simulink model "CRH2forBenchmark_Copy"  (R2014a)
settings: Solver=ode3  StartTime=0.0  StopTime=1  FixedStep=1e-5  RelTol=1e-3
PostLoadFcn:
  | , if any(exist('dsrtsu_mdlpostloadfcn', 'file') == [2, 3, 6]), try dsrtsu_mdlpostloadfcn('Execute', bdroot); catch fprintf('Error in PostLoadFcn (dsrtsu_mdlpostloadfcn) for model "%s":\n %s\n', bdroot, lasterr); end, end,
values from neighbouring files (symbols this model uses):
  Cd = 0.016    [CRH2forBenchmark.mat]
  Lm = 0.032848    [CRH2forBenchmark.mat]
  Ln = 0.002    [CRH2forBenchmark.mat]
  Lr = 0.034142    [CRH2forBenchmark.mat]
  Ls = 0.0342654    [CRH2forBenchmark.mat]
  np = 2    [CRH2forBenchmark.mat]
  Rd = 6000    [CRH2forBenchmark.mat]
  Rn = 0.2    [CRH2forBenchmark.mat]
  Rr = 0.146    [CRH2forBenchmark.mat]
  Rs = 0.144    [CRH2forBenchmark.mat]
  ts = 1e-05    [CRH2forBenchmark.mat]
undefined symbols (not defined in the file): J, KIM, KIT, KPM, KPT, phir, Ts, Vge
libraries: simulink x20
(part 2 of 5)

== system CRH2forBenchmark_Copy/Benchmark/MFI1 ==
  MFI1 : Subsystem  mask(MFI){FaultType=Normal, FaultInjectionTime=1, FS=[128.7,0.038], Severity1=0.5, Severity3=0.2, Severity2=0.2, BearingFP=[1,8,25,25,65,0,20], NoiseSelec=off, NoiseFault=[0.001 1e-5 23341], AddMux=Add}
      mask prompts: FaultType "Fault Type"; FaultInjectionTime "Fault Injection Time(Step time)"; FS "Fundamental Frequency and Slip Ratio[f1 S]"; Severity1 "Mechanical Fault Severity (0-1)(Bar Broken fault;End Link Fault;Bearing Fault)"; Severity3 "Electrical Fault Severity(0-1)(Air Gap Eccentricity Fault)"; Severity2 "Insulation Fault Severity(0-1)(Inter-turn Short Circuit Fault)"; BearingFP "Bearing Fault Parameters [T Z fr d D a fcage]"; NoiseSelec "Noise Disturbance"; NoiseFault "Noise Disturbance(Noise power,Sample time,Seed)"; AddMux "Add or Mux(outside signal)"
      mask help:
      | Machine Fault Injector (MFI)
      | 1.Fault Injection Time:Set the parameter of Fault-Inject Time;
      | 2.Fundamental Frequency and Slip Ratio[f1 S]:The current frequency of motor stator and the motor Slip Ratio.
      | 3.Mechanical Fault Severity (0-1)(Bar Broken fault;End Link Fault;Bearing Fault):Mechanical Failure factor denotes the fault severity（0-1）.Three types of Mechanical faults are taken into consideration;
      | 4.Electrical Fault Severity(0-1)(Air Gap Eccentricity Fault):Electrical Failure factor denotes the fault severity（0-1）.
      | 5.Insulation Fault Severity(0-1)(Inter-turn Short Circuit Fault):Insulation Failure factor denotes the fault severity（0-1）.
      | 6.Bearing Fault Parameters [T Z fr d D a fcage]: The value of S are constraint to [1,2,3], T=1 represents the outer ring fault,T=2 represents the bearing inner race fault, T=3 represents rolling body defect fault;Z is the number of bearing rollers;fr is motor bearing frequency;d is the bearing diameter of the rolling body;D is bearing section diameter;a is contact angle;fcage is cage rotation frequency.
      mask TypeOptions FaultType: Normal | Bar Broken Fault | Inter-turn Short Circuit Fault | Air Gap Eccentricity Fault | End Link Fault | Bearing Fault | Outside Signal
      mask TypeOptions AddMux: Add | Mux | Replace
      mask Display: fprintf('Motor Fault Injection')
  MFI2 : Subsystem  mask(MFI){FaultType=Normal, FaultInjectionTime=1, FS=[128.7,0.038], Severity1=0.5, Severity3=0.2, Severity2=0.2, BearingFP=[1,8,25,25,65,0,20], NoiseSelec=off, NoiseFault=[0.001 1e-5 23341], AddMux=Add}
      mask prompts: FaultType "Fault Type"; FaultInjectionTime "Fault Injection Time(Step time)"; FS "Fundamental Frequency and Slip Ratio[f1 S]"; Severity1 "Mechanical Fault Severity (0-1)(Bar Broken fault;End Link Fault;Bearing Fault)"; Severity3 "Electrical Fault Severity(0-1)(Air Gap Eccentricity Fault)"; Severity2 "Insulation Fault Severity(0-1)(Inter-turn Short Circuit Fault)"; BearingFP "Bearing Fault Parameters [T Z fr d D a fcage]"; NoiseSelec "Noise Disturbance"; NoiseFault "Noise Disturbance(Noise power,Sample time,Seed)"; AddMux "Add or Mux(outside signal)"
      mask help:
      | Machine Fault Injector (MFI)
      | 1.Fault Injection Time:Set the parameter of Fault-Inject Time;
      | 2.Fundamental Frequency and Slip Ratio[f1 S]:The current frequency of motor stator and the motor Slip Ratio.
      | 3.Mechanical Fault Severity (0-1)(Bar Broken fault;End Link Fault;Bearing Fault):Mechanical Failure factor denotes the fault severity（0-1）.Three types of Mechanical faults are taken into consideration;
      | 4.Electrical Fault Severity(0-1)(Air Gap Eccentricity Fault):Electrical Failure factor denotes the fault severity（0-1）.
      | 5.Insulation Fault Severity(0-1)(Inter-turn Short Circuit Fault):Insulation Failure factor denotes the fault severity（0-1）.
      | 6.Bearing Fault Parameters [T Z fr d D a fcage]: The value of S are constraint to [1,2,3], T=1 represents the outer ring fault,T=2 represents the bearing inner race fault, T=3 represents rolling body defect fault;Z is the number of bearing rollers;fr is motor bearing frequency;d is the bearing diameter of the rolling body;D is bearing section diameter;a is contact angle;fcage is cage rotation frequency.
      mask TypeOptions FaultType: Normal | Bar Broken Fault | Inter-turn Short Circuit Fault | Air Gap Eccentricity Fault | End Link Fault | Bearing Fault | Outside Signal
      mask TypeOptions AddMux: Add | Mux | Replace
      mask Display: fprintf('Motor Fault Injection')
  MFI3 : Subsystem  mask(MFI){FaultType=Normal, FaultInjectionTime=1, FS=[128.7,0.038], Severity1=0.5, Severity3=0.2, Severity2=0.2, BearingFP=[1,8,25,25,65,0,20], NoiseSelec=off, NoiseFault=[0.001 1e-5 23341], AddMux=Add}
      mask prompts: FaultType "Fault Type"; FaultInjectionTime "Fault Injection Time(Step time)"; FS "Fundamental Frequency and Slip Ratio[f1 S]"; Severity1 "Mechanical Fault Severity (0-1)(Bar Broken fault;End Link Fault;Bearing Fault)"; Severity3 "Electrical Fault Severity(0-1)(Air Gap Eccentricity Fault)"; Severity2 "Insulation Fault Severity(0-1)(Inter-turn Short Circuit Fault)"; BearingFP "Bearing Fault Parameters [T Z fr d D a fcage]"; NoiseSelec "Noise Disturbance"; NoiseFault "Noise Disturbance(Noise power,Sample time,Seed)"; AddMux "Add or Mux(outside signal)"
      mask help:
      | Machine Fault Injector (MFI)
      | 1.Fault Injection Time:Set the parameter of Fault-Inject Time;
      | 2.Fundamental Frequency and Slip Ratio[f1 S]:The current frequency of motor stator and the motor Slip Ratio.
      | 3.Mechanical Fault Severity (0-1)(Bar Broken fault;End Link Fault;Bearing Fault):Mechanical Failure factor denotes the fault severity（0-1）.Three types of Mechanical faults are taken into consideration;
      | 4.Electrical Fault Severity(0-1)(Air Gap Eccentricity Fault):Electrical Failure factor denotes the fault severity（0-1）.
      | 5.Insulation Fault Severity(0-1)(Inter-turn Short Circuit Fault):Insulation Failure factor denotes the fault severity（0-1）.
      | 6.Bearing Fault Parameters [T Z fr d D a fcage]: The value of S are constraint to [1,2,3], T=1 represents the outer ring fault,T=2 represents the bearing inner race fault, T=3 represents rolling body defect fault;Z is the number of bearing rollers;fr is motor bearing frequency;d is the bearing diameter of the rolling body;D is bearing section diameter;a is contact angle;fcage is cage rotation frequency.
      mask TypeOptions FaultType: Normal | Bar Broken Fault | Inter-turn Short Circuit Fault | Air Gap Eccentricity Fault | End Link Fault | Bearing Fault | Outside Signal
      mask TypeOptions AddMux: Add | Mux | Replace
      mask Display: fprintf('Motor Fault Injection')
  MFI4 : Subsystem  mask(MFI){FaultType=Normal, FaultInjectionTime=1, FS=[128.7,0.038], Severity1=0.5, Severity3=0.2, Severity2=0.2, BearingFP=[1,8,25,25,65,0,20], NoiseSelec=off, NoiseFault=[0.001 1e-5 23341], AddMux=Add}
      mask prompts: FaultType "Fault Type"; FaultInjectionTime "Fault Injection Time(Step time)"; FS "Fundamental Frequency and Slip Ratio[f1 S]"; Severity1 "Mechanical Fault Severity (0-1)(Bar Broken fault;End Link Fault;Bearing Fault)"; Severity3 "Electrical Fault Severity(0-1)(Air Gap Eccentricity Fault)"; Severity2 "Insulation Fault Severity(0-1)(Inter-turn Short Circuit Fault)"; BearingFP "Bearing Fault Parameters [T Z fr d D a fcage]"; NoiseSelec "Noise Disturbance"; NoiseFault "Noise Disturbance(Noise power,Sample time,Seed)"; AddMux "Add or Mux(outside signal)"
      mask help:
      | Machine Fault Injector (MFI)
      | 1.Fault Injection Time:Set the parameter of Fault-Inject Time;
      | 2.Fundamental Frequency and Slip Ratio[f1 S]:The current frequency of motor stator and the motor Slip Ratio.
      | 3.Mechanical Fault Severity (0-1)(Bar Broken fault;End Link Fault;Bearing Fault):Mechanical Failure factor denotes the fault severity（0-1）.Three types of Mechanical faults are taken into consideration;
      | 4.Electrical Fault Severity(0-1)(Air Gap Eccentricity Fault):Electrical Failure factor denotes the fault severity（0-1）.
      | 5.Insulation Fault Severity(0-1)(Inter-turn Short Circuit Fault):Insulation Failure factor denotes the fault severity（0-1）.
      | 6.Bearing Fault Parameters [T Z fr d D a fcage]: The value of S are constraint to [1,2,3], T=1 represents the outer ring fault,T=2 represents the bearing inner race fault, T=3 represents rolling body defect fault;Z is the number of bearing rollers;fr is motor bearing frequency;d is the bearing diameter of the rolling body;D is bearing section diameter;a is contact angle;fcage is cage rotation frequency.
      mask TypeOptions FaultType: Normal | Bar Broken Fault | Inter-turn Short Circuit Fault | Air Gap Eccentricity Fault | End Link Fault | Bearing Fault | Outside Signal
      mask TypeOptions AddMux: Add | Mux | Replace
      mask Display: fprintf('Motor Fault Injection')
  MFI5 : Subsystem  mask(MFI){FaultType=Normal, FaultInjectionTime=1, FS=[128.7,0.038], Severity1=0.5, Severity3=0.2, Severity2=0.2, BearingFP=[1,8,25,25,65,0,20], NoiseSelec=off, NoiseFault=[0.001 1e-5 23341], AddMux=Add}
      mask prompts: FaultType "Fault Type"; FaultInjectionTime "Fault Injection Time(Step time)"; FS "Fundamental Frequency and Slip Ratio[f1 S]"; Severity1 "Mechanical Fault Severity (0-1)(Bar Broken fault;End Link Fault;Bearing Fault)"; Severity3 "Electrical Fault Severity(0-1)(Air Gap Eccentricity Fault)"; Severity2 "Insulation Fault Severity(0-1)(Inter-turn Short Circuit Fault)"; BearingFP "Bearing Fault Parameters [T Z fr d D a fcage]"; NoiseSelec "Noise Disturbance"; NoiseFault "Noise Disturbance(Noise power,Sample time,Seed)"; AddMux "Add or Mux(outside signal)"
      mask help:
      | Machine Fault Injector (MFI)
      | 1.Fault Injection Time:Set the parameter of Fault-Inject Time;
      | 2.Fundamental Frequency and Slip Ratio[f1 S]:The current frequency of motor stator and the motor Slip Ratio.
      | 3.Mechanical Fault Severity (0-1)(Bar Broken fault;End Link Fault;Bearing Fault):Mechanical Failure factor denotes the fault severity（0-1）.Three types of Mechanical faults are taken into consideration;
      | 4.Electrical Fault Severity(0-1)(Air Gap Eccentricity Fault):Electrical Failure factor denotes the fault severity（0-1）.
      | 5.Insulation Fault Severity(0-1)(Inter-turn Short Circuit Fault):Insulation Failure factor denotes the fault severity（0-1）.
      | 6.Bearing Fault Parameters [T Z fr d D a fcage]: The value of S are constraint to [1,2,3], T=1 represents the outer ring fault,T=2 represents the bearing inner race fault, T=3 represents rolling body defect fault;Z is the number of bearing rollers;fr is motor bearing frequency;d is the bearing diameter of the rolling body;D is bearing section diameter;a is contact angle;fcage is cage rotation frequency.
      mask TypeOptions FaultType: Normal | Bar Broken Fault | Inter-turn Short Circuit Fault | Air Gap Eccentricity Fault | End Link Fault | Bearing Fault | Outside Signal
      mask TypeOptions AddMux: Add | Mux | Replace
      mask Display: fprintf('Motor Fault Injection')
  MFI6 : Subsystem  mask(MFI){FaultType=Normal, FaultInjectionTime=1, FS=[128.7,0.038], Severity1=0.5, Severity3=0.2, Severity2=0.2, BearingFP=[1,8,25,25,65,0,20], NoiseSelec=off, NoiseFault=[0.001 1e-5 23341], AddMux=Add}
      mask prompts: FaultType "Fault Type"; FaultInjectionTime "Fault Injection Time(Step time)"; FS "Fundamental Frequency and Slip Ratio[f1 S]"; Severity1 "Mechanical Fault Severity (0-1)(Bar Broken fault;End Link Fault;Bearing Fault)"; Severity3 "Electrical Fault Severity(0-1)(Air Gap Eccentricity Fault)"; Severity2 "Insulation Fault Severity(0-1)(Inter-turn Short Circuit Fault)"; BearingFP "Bearing Fault Parameters [T Z fr d D a fcage]"; NoiseSelec "Noise Disturbance"; NoiseFault "Noise Disturbance(Noise power,Sample time,Seed)"; AddMux "Add or Mux(outside signal)"
      mask help:
      | Machine Fault Injector (MFI)
      | 1.Fault Injection Time:Set the parameter of Fault-Inject Time;
      | 2.Fundamental Frequency and Slip Ratio[f1 S]:The current frequency of motor stator and the motor Slip Ratio.
      | 3.Mechanical Fault Severity (0-1)(Bar Broken fault;End Link Fault;Bearing Fault):Mechanical Failure factor denotes the fault severity（0-1）.Three types of Mechanical faults are taken into consideration;
      | 4.Electrical Fault Severity(0-1)(Air Gap Eccentricity Fault):Electrical Failure factor denotes the fault severity（0-1）.
      | 5.Insulation Fault Severity(0-1)(Inter-turn Short Circuit Fault):Insulation Failure factor denotes the fault severity（0-1）.
      | 6.Bearing Fault Parameters [T Z fr d D a fcage]: The value of S are constraint to [1,2,3], T=1 represents the outer ring fault,T=2 represents the bearing inner race fault, T=3 represents rolling body defect fault;Z is the number of bearing rollers;fr is motor bearing frequency;d is the bearing diameter of the rolling body;D is bearing section diameter;a is contact angle;fcage is cage rotation frequency.
      mask TypeOptions FaultType: Normal | Bar Broken Fault | Inter-turn Short Circuit Fault | Air Gap Eccentricity Fault | End Link Fault | Bearing Fault | Outside Signal
      mask TypeOptions AddMux: Add | Mux | Replace
      mask Display: fprintf('Motor Fault Injection')

== system CRH2forBenchmark_Copy/Benchmark/SFI1 ==
  Normal : Inport
  Outside Signal : Inport  Port=2
  Subsystem : Subsystem
  Out : Outport
  wires:
  Normal/1 -> Subsystem/1(Normal)
  Outside Signal/1 -> Subsystem/2(Outside Signal)
  Subsystem/1(Out) -> Out/1

== system CRH2forBenchmark_Copy/Benchmark/SFI2 ==
  Normal : Inport
  Outside Signal : Inport  Port=2
  Subsystem : Subsystem
  Out : Outport
  wires:
  Normal/1 -> Subsystem/1(Normal)
  Outside Signal/1 -> Subsystem/2(Outside Signal)
  Subsystem/1(Out) -> Out/1

== system CRH2forBenchmark_Copy/Benchmark/TFI1 ==
  Nomal : Inport
  Outside Signal : Inport  Port=2
  TFI1Sub : Subsystem
  Out : Outport
  wires:
  Nomal/1 -> TFI1Sub/1(Nomal)
  Outside Signal/1 -> TFI1Sub/2(Outside Signal)
  TFI1Sub/1(Out) -> Out/1

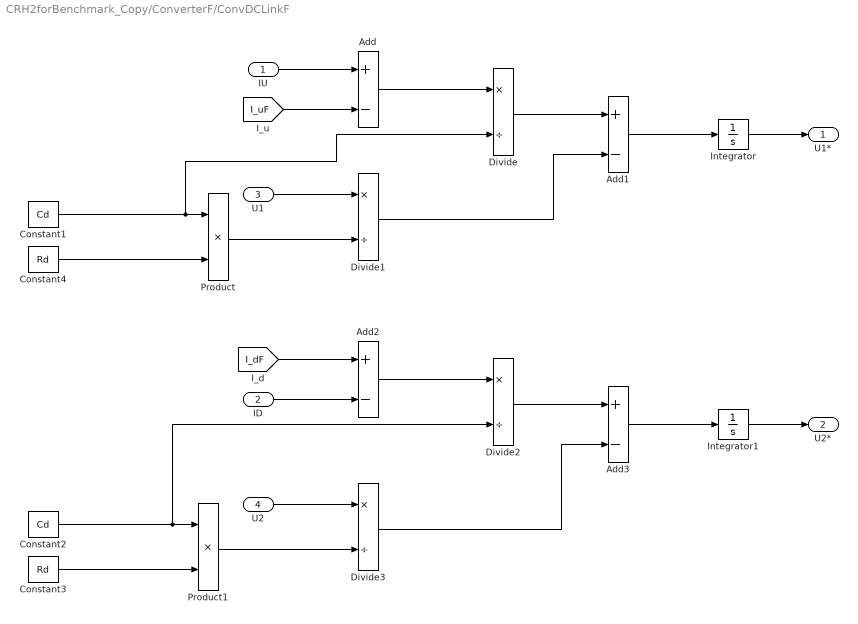
== system CRH2forBenchmark_Copy/ConverterF/ConvDCLinkF ==
  IU : Inport
  ID : Inport  Port=2
  U1 : Inport  Port=3
  U2 : Inport  Port=4
  Add{,1..3} (4 alike) : Sum  Inputs=+-  SampleTime=ts
  Constant1 : Constant  Value=Cd
  Constant2 : Constant  Value=Cd
  Constant3 : Constant  Value=Rd
  Constant4 : Constant  Value=Rd
  Divide{,1..3} (4 alike) : Product  Inputs=*/
  Integrator : Integrator
  Integrator1 : Integrator
  Product : Product  SampleTime=ts
  Product1 : Product  SampleTime=ts
  U1* : Outport
  U2* : Outport  Port=2
  wires:
  Add3/1 -> Integrator1/1
  Divide3/1 -> Add3/2
  Divide2/1 -> Add3/1
  U2/1 -> Divide3/1
  Product1/1 -> Divide3/2
  Add2/1 -> Divide2/1
  Constant2/1 -> Divide2/2, Product1/1
  [I_dF] -> Add2/1
  ID/1 -> Add2/2
  Add1/1 -> Integrator/1
  Divide1/1 -> Add1/2
  Divide/1 -> Add1/1
  U1/1 -> Divide1/1
  Constant1/1 -> Product/1, Divide/2
  Add/1 -> Divide/1
  [I_uF] -> Add/2
  IU/1 -> Add/1
  Integrator/1 -> U1*/1
  Integrator1/1 -> U2*/1
  Product/1 -> Divide1/2
  Constant4/1 -> Product/2
  Constant3/1 -> Product1/2

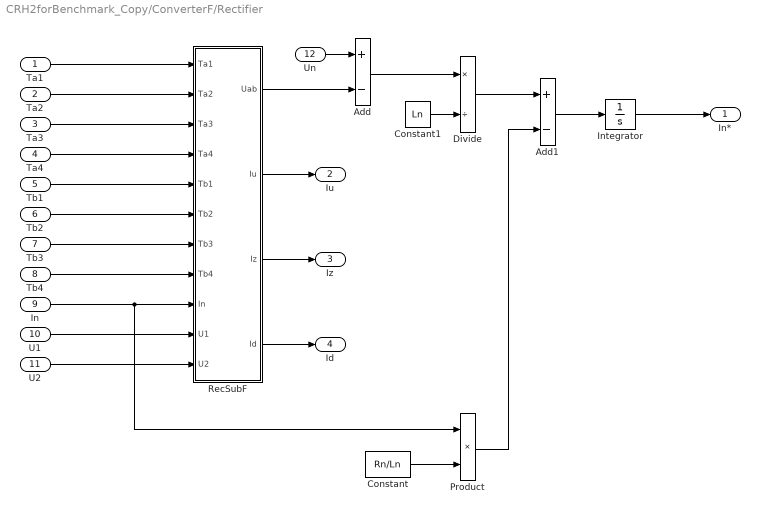
== system CRH2forBenchmark_Copy/ConverterF/Rectifier ==
  Ta1 : Inport
  Ta2 : Inport  Port=2
  Ta3 : Inport  Port=3
  Ta4 : Inport  Port=4
  Tb1 : Inport  Port=5
  Tb2 : Inport  Port=6
  Tb3 : Inport  Port=7
  Tb4 : Inport  Port=8
  In : Inport  Port=9
  U1 : Inport  Port=10
  U2 : Inport  Port=11
  Un : Inport  Port=12
  Add : Sum  Inputs=+-  SampleTime=ts
  Add1 : Sum  Inputs=+-  SampleTime=ts
  Constant : Constant  Value=Rn/Ln
  Constant1 : Constant  Value=Ln
  Divide : Product  Inputs=*/  SampleTime=ts
  Integrator : Integrator
  Product : Product  SampleTime=ts
  RecSubF : Subsystem
  In* : Outport
  Iu : Outport  Port=2
  Iz : Outport  Port=3
  Id : Outport  Port=4
  wires:
  RecSubF/4(Id) -> Id/1
  RecSubF/3(Iz) -> Iz/1
  RecSubF/2(Iu) -> Iu/1
  Tb2/1 -> RecSubF/6(Tb2)
  Ta3/1 -> RecSubF/3(Ta3)
  Un/1 -> Add/1
  Tb1/1 -> RecSubF/5(Tb1)
  Tb4/1 -> RecSubF/8(Tb4)
  Tb3/1 -> RecSubF/7(Tb3)
  In/1 -> Product/1, RecSubF/9(In)
  Ta4/1 -> RecSubF/4(Ta4)
  Ta2/1 -> RecSubF/2(Ta2)
  U2/1 -> RecSubF/11(U2)
  Integrator/1 -> In*/1
  Divide/1 -> Add1/1
  U1/1 -> RecSubF/10(U1)
  Constant/1 -> Product/2
  RecSubF/1(Uab) -> Add/2
  Ta1/1 -> RecSubF/1(Ta1)
  Add1/1 -> Integrator/1
  Product/1 -> Add1/2
  Constant1/1 -> Divide/2
  Add/1 -> Divide/1

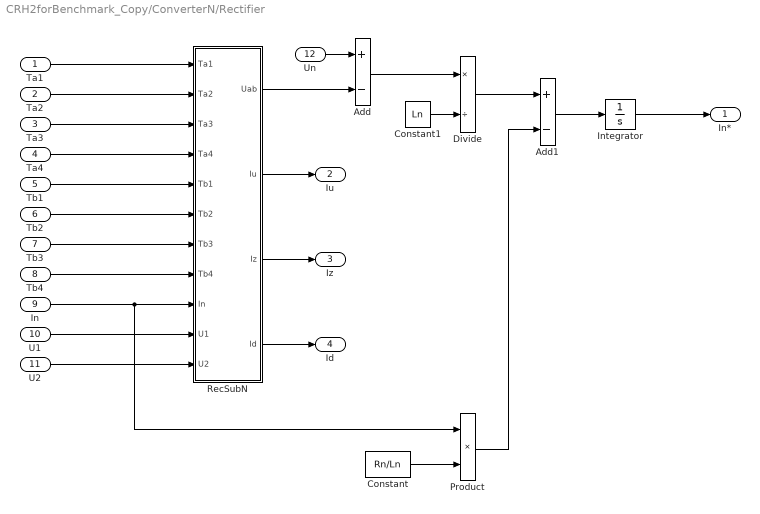
== system CRH2forBenchmark_Copy/ConverterN/Rectifier ==
  Ta1 : Inport
  Ta2 : Inport  Port=2
  Ta3 : Inport  Port=3
  Ta4 : Inport  Port=4
  Tb1 : Inport  Port=5
  Tb2 : Inport  Port=6
  Tb3 : Inport  Port=7
  Tb4 : Inport  Port=8
  In : Inport  Port=9
  U1 : Inport  Port=10
  U2 : Inport  Port=11
  Un : Inport  Port=12
  Add : Sum  Inputs=+-  SampleTime=ts
  Add1 : Sum  Inputs=+-  SampleTime=ts
  Constant : Constant  Value=Rn/Ln
  Constant1 : Constant  Value=Ln
  Divide : Product  Inputs=*/  SampleTime=ts
  Integrator : Integrator
  Product : Product  SampleTime=ts
  RecSubN : Subsystem
  In* : Outport
  Iu : Outport  Port=2
  Iz : Outport  Port=3
  Id : Outport  Port=4
  wires:
  Add/1 -> Divide/1
  Constant1/1 -> Divide/2
  Product/1 -> Add1/2
  Add1/1 -> Integrator/1
  Ta1/1 -> RecSubN/1(Ta1)
  RecSubN/1(Uab) -> Add/2
  Constant/1 -> Product/2
  U1/1 -> RecSubN/10(U1)
  Divide/1 -> Add1/1
  Integrator/1 -> In*/1
  U2/1 -> RecSubN/11(U2)
  Ta2/1 -> RecSubN/2(Ta2)
  Ta4/1 -> RecSubN/4(Ta4)
  In/1 -> RecSubN/9(In), Product/1
  Tb3/1 -> RecSubN/7(Tb3)
  Tb4/1 -> RecSubN/8(Tb4)
  Tb1/1 -> RecSubN/5(Tb1)
  Un/1 -> Add/1
  Ta3/1 -> RecSubN/3(Ta3)
  Tb2/1 -> RecSubN/6(Tb2)
  RecSubN/2(Iu) -> Iu/1
  RecSubN/3(Iz) -> Iz/1
  RecSubN/4(Id) -> Id/1

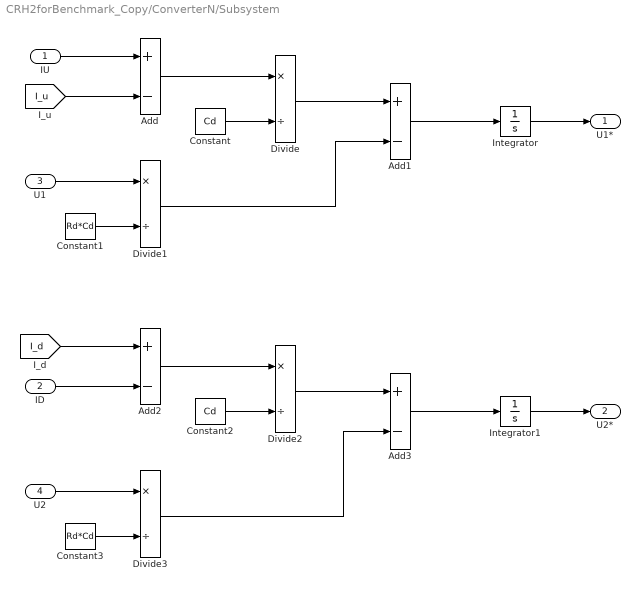
== system CRH2forBenchmark_Copy/ConverterN/Subsystem ==
  IU : Inport
  ID : Inport  Port=2
  U1 : Inport  Port=3
  U2 : Inport  Port=4
  Add{,1..3} (4 alike) : Sum  Inputs=+-  SampleTime=ts
  Constant : Constant  Value=Cd
  Constant1 : Constant  Value=Rd*Cd
  Constant2 : Constant  Value=Cd
  Constant3 : Constant  Value=Rd*Cd
  Divide{,1..3} (4 alike) : Product  Inputs=*/
  Integrator : Integrator
  Integrator1 : Integrator
  U1* : Outport
  U2* : Outport  Port=2
  wires:
  Integrator1/1 -> U2*/1
  Integrator/1 -> U1*/1
  IU/1 -> Add/1
  [I_u] -> Add/2
  Add/1 -> Divide/1
  Constant/1 -> Divide/2
  U1/1 -> Divide1/1
  Constant1/1 -> Divide1/2
  Divide/1 -> Add1/1
  Divide1/1 -> Add1/2
  Add1/1 -> Integrator/1
  ID/1 -> Add2/2
  [I_d] -> Add2/1
  Constant2/1 -> Divide2/2
  Add2/1 -> Divide2/1
  Constant3/1 -> Divide3/2
  U2/1 -> Divide3/1
  Divide2/1 -> Add3/1
  Divide3/1 -> Add3/2
  Add3/1 -> Integrator1/1

== system CRH2forBenchmark_Copy/DCU1/__InputSSForSFun__ ==
  Commander : Inport
  __UniqueOutportName__1__ : Outport
  __UniqueOutportName__2__ : Outport  Port=2
  __UniqueOutportName__3__ : Outport  Port=3
  __UniqueOutportName__4__ : Outport  Port=4
  __UniqueOutportName__5__ : Outport  Port=5
  __UniqueOutportName__6__ : Outport  Port=6
  __UniqueOutportName__7__ : Outport  Port=7
  __UniqueOutportName__8__ : Outport  Port=8
  __UniqueOutportName__9__ : Outport  Port=9
  wires:
  [w0] -> __UniqueOutportName__9__/1
  [Isabc0] -> __UniqueOutportName__8__/1
  [TL] -> __UniqueOutportName__7__/1
  [Ucd1] -> __UniqueOutportName__6__/1
  [In] -> __UniqueOutportName__5__/1
  [Un] -> __UniqueOutportName__4__/1
  [Ucd2] -> __UniqueOutportName__3__/1
  [Id] -> __UniqueOutportName__2__/1
  Commander/1 -> __UniqueOutportName__1__/1

== system CRH2forBenchmark_Copy/DCU1/__OutputSSForSFun__ ==
  __UniqueInportName__1__ : Inport
  __UniqueInportName__2__ : Inport  Port=2
  SPWM1 : Outport
  SPWM : Outport  Port=2
  wires:
  __UniqueInportName__2__/1 -> SPWM/1
  __UniqueInportName__1__/1 -> SPWM1/1

== system CRH2forBenchmark_Copy/DCU2/__InputSSForSFun__ ==
  Commander : Inport
  __UniqueOutportName__1__ : Outport
  __UniqueOutportName__2__ : Outport  Port=2
  __UniqueOutportName__3__ : Outport  Port=3
  __UniqueOutportName__4__ : Outport  Port=4
  __UniqueOutportName__5__ : Outport  Port=5
  __UniqueOutportName__6__ : Outport  Port=6
  __UniqueOutportName__7__ : Outport  Port=7
  __UniqueOutportName__8__ : Outport  Port=8
  __UniqueOutportName__9__ : Outport  Port=9
  wires:
  Commander/1 -> __UniqueOutportName__1__/1
  [IdF] -> __UniqueOutportName__2__/1
  [Ucd2F] -> __UniqueOutportName__3__/1
  [UnF] -> __UniqueOutportName__4__/1
  [InF] -> __UniqueOutportName__5__/1
  [Ucd1F] -> __UniqueOutportName__6__/1
  [TLF] -> __UniqueOutportName__7__/1
  [Isabc0F] -> __UniqueOutportName__8__/1
  [w0F] -> __UniqueOutportName__9__/1

== system CRH2forBenchmark_Copy/DCU2/__OutputSSForSFun__ ==
  __UniqueInportName__1__ : Inport
  __UniqueInportName__2__ : Inport  Port=2
  SPWM1 : Outport
  SPWM : Outport  Port=2
  wires:
  __UniqueInportName__1__/1 -> SPWM1/1
  __UniqueInportName__2__/1 -> SPWM/1

== system CRH2forBenchmark_Copy/IntermediateDClinkF/__InputSSForSFun__ ==
  In1 : Inport
  In2 : Inport  Port=2
  In3 : Inport  Port=3
  In4 : Inport  Port=4
  __UniqueOutportName__1__ : Outport
  __UniqueOutportName__2__ : Outport  Port=2
  __UniqueOutportName__3__ : Outport  Port=3
  __UniqueOutportName__4__ : Outport  Port=4
  wires:
  In1/1 -> __UniqueOutportName__1__/1
  In2/1 -> __UniqueOutportName__2__/1
  In3/1 -> __UniqueOutportName__3__/1
  In4/1 -> __UniqueOutportName__4__/1

== system CRH2forBenchmark_Copy/IntermediateDClinkF/__OutputSSForSFun__ ==
  __UniqueInportName__1__ : Inport
  __UniqueInportName__2__ : Inport  Port=2
  __UniqueInportName__3__ : Inport  Port=3
  Out1 : Outport
  Out4 : Outport  Port=2
  Out7 : Outport  Port=3
  wires:
  __UniqueInportName__1__/1 -> Out1/1
  __UniqueInportName__2__/1 -> Out4/1
  __UniqueInportName__3__/1 -> Out7/1

== system CRH2forBenchmark_Copy/IntermediateDClinkN/__InputSSForSFun__ ==
  In1 : Inport
  In2 : Inport  Port=2
  In3 : Inport  Port=3
  In4 : Inport  Port=4
  __UniqueOutportName__1__ : Outport
  __UniqueOutportName__2__ : Outport  Port=2
  __UniqueOutportName__3__ : Outport  Port=3
  __UniqueOutportName__4__ : Outport  Port=4
  wires:
  In1/1 -> __UniqueOutportName__1__/1
  In2/1 -> __UniqueOutportName__2__/1
  In3/1 -> __UniqueOutportName__3__/1
  In4/1 -> __UniqueOutportName__4__/1

== system CRH2forBenchmark_Copy/IntermediateDClinkN/__OutputSSForSFun__ ==
  __UniqueInportName__1__ : Inport
  __UniqueInportName__2__ : Inport  Port=2
  __UniqueInportName__3__ : Inport  Port=3
  Out1 : Outport
  Out4 : Outport  Port=2
  Out7 : Outport  Port=3
  wires:
  __UniqueInportName__1__/1 -> Out1/1
  __UniqueInportName__2__/1 -> Out4/1
  __UniqueInportName__3__/1 -> Out7/1

== system CRH2forBenchmark_Copy/InverterF/InverterTuF ==
  Tu1 : Inport
  Tu2 : Inport  Port=2
  Tu3 : Inport  Port=3
  Tu4 : Inport  Port=4
  Ia : Inport  Port=5
  U1 : Inport  Port=6
  U2 : Inport  Port=7
  InverterTuF_sfcn : S-Function  FunctionName=InverterTuF_sf  SFunctionModules=""  EnableBusSupport=off  mask{rtw_sf_name=InverterTuF_sf, showVar=off}
      mask prompts: rtw_sf_name "Simulink:masks:GenSFuncName_MP"; showVar "Simulink:masks:GenSFuncShowModuleList_MP"
      mask help: Simulink:masks:GenSFuncDesc_MD
      mask init: same as CRH2forBenchmark_Copy/DCU1/DCU1_sfcn
      settings: CopyFcn=|
      | if ~strcmp(get_param(gcb,'Linkstatus'),'none') && ...
      | ~strcmp(get_param(gcb,'Linkstatus'),'implicit')
      |   set_param(gcb,'LinkStatus','none');
      | end
      mask Help: eval('feval(''rtwprivate'',''rtwhelpview'',''rtw_sfcn_block'')');
      mask Display:
      | port_label('input',1,'Tu1');
      | port_label('input',2,'Tu2');
      | port_label('input',3,'Tu3');
      | port_label('input',4,'Tu4');
      | port_label('input',5,'Ia');
      | port_label('input',6,'U1');
      | port_label('input',7,'U2');
      | port_label('output',1,'Iu');
      | port_label('output',2,'Iz');
      | port_label('output',3,'Id');
      | port_label('output',4,'Vu');
  __InputSSForSFun__ : Subsystem
  __OutputSSForSFun__ : Subsystem
  Iu : Outport
  Iz : Outport  Port=2
  Id : Outport  Port=3
  Vu : Outport  Port=4
  wires:
  Tu1/1 -> __InputSSForSFun__/1(Tu1)
  Tu2/1 -> __InputSSForSFun__/2(Tu2)
  Tu3/1 -> __InputSSForSFun__/3(Tu3)
  Tu4/1 -> __InputSSForSFun__/4(Tu4)
  Ia/1 -> __InputSSForSFun__/5(Ia)
  U1/1 -> __InputSSForSFun__/6(U1)
  U2/1 -> __InputSSForSFun__/7(U2)
  __InputSSForSFun__/1(__UniqueOutportName__1__) -> InverterTuF_sfcn/1
  __InputSSForSFun__/2(__UniqueOutportName__2__) -> InverterTuF_sfcn/2
  __InputSSForSFun__/3(__UniqueOutportName__3__) -> InverterTuF_sfcn/3
  __InputSSForSFun__/4(__UniqueOutportName__4__) -> InverterTuF_sfcn/4
  __InputSSForSFun__/5(__UniqueOutportName__5__) -> InverterTuF_sfcn/5
  __InputSSForSFun__/6(__UniqueOutportName__6__) -> InverterTuF_sfcn/6
  __InputSSForSFun__/7(__UniqueOutportName__7__) -> InverterTuF_sfcn/7
  InverterTuF_sfcn/1 -> __OutputSSForSFun__/1(__UniqueInportName__1__)
  InverterTuF_sfcn/2 -> __OutputSSForSFun__/2(__UniqueInportName__2__)
  InverterTuF_sfcn/3 -> __OutputSSForSFun__/3(__UniqueInportName__3__)
  InverterTuF_sfcn/4 -> __OutputSSForSFun__/4(__UniqueInportName__4__)
  __OutputSSForSFun__/1(Iu) -> Iu/1
  __OutputSSForSFun__/2(Iz) -> Iz/1
  __OutputSSForSFun__/3(Id) -> Id/1
  __OutputSSForSFun__/4(Vu) -> Vu/1

== system CRH2forBenchmark_Copy/InverterF/InverterTvF ==
  Tv1 : Inport
  Tv2 : Inport  Port=2
  Tv3 : Inport  Port=3
  Tv4 : Inport  Port=4
  Ib : Inport  Port=5
  U1 : Inport  Port=6
  U2 : Inport  Port=7
  InverterTvF_sfcn : S-Function  FunctionName=InverterTvF_sf  SFunctionModules=""  EnableBusSupport=off  mask{rtw_sf_name=InverterTvF_sf, showVar=off}
      mask prompts: rtw_sf_name "Simulink:masks:GenSFuncName_MP"; showVar "Simulink:masks:GenSFuncShowModuleList_MP"
      mask help: Simulink:masks:GenSFuncDesc_MD
      mask init: same as CRH2forBenchmark_Copy/DCU1/DCU1_sfcn
      settings: CopyFcn=|
      | if ~strcmp(get_param(gcb,'Linkstatus'),'none') && ...
      | ~strcmp(get_param(gcb,'Linkstatus'),'implicit')
      |   set_param(gcb,'LinkStatus','none');
      | end
      mask Help: eval('feval(''rtwprivate'',''rtwhelpview'',''rtw_sfcn_block'')');
      mask Display:
      | port_label('input',1,'Tv1');
      | port_label('input',2,'Tv2');
      | port_label('input',3,'Tv3');
      | port_label('input',4,'Tv4');
      | port_label('input',5,'Ib');
      | port_label('input',6,'U1');
      | port_label('input',7,'U2');
      | port_label('output',1,'Iu');
      | port_label('output',2,'Iz');
      | port_label('output',3,'Id');
      | port_label('output',4,'Vv');
  __InputSSForSFun__ : Subsystem
  __OutputSSForSFun__ : Subsystem
  Iu : Outport
  Iz : Outport  Port=2
  Id : Outport  Port=3
  Vv : Outport  Port=4
  wires:
  Tv1/1 -> __InputSSForSFun__/1(Tv1)
  Tv2/1 -> __InputSSForSFun__/2(Tv2)
  Tv3/1 -> __InputSSForSFun__/3(Tv3)
  Tv4/1 -> __InputSSForSFun__/4(Tv4)
  Ib/1 -> __InputSSForSFun__/5(Ib)
  U1/1 -> __InputSSForSFun__/6(U1)
  U2/1 -> __InputSSForSFun__/7(U2)
  __InputSSForSFun__/1(__UniqueOutportName__1__) -> InverterTvF_sfcn/1
  __InputSSForSFun__/2(__UniqueOutportName__2__) -> InverterTvF_sfcn/2
  __InputSSForSFun__/3(__UniqueOutportName__3__) -> InverterTvF_sfcn/3
  __InputSSForSFun__/4(__UniqueOutportName__4__) -> InverterTvF_sfcn/4
  __InputSSForSFun__/5(__UniqueOutportName__5__) -> InverterTvF_sfcn/5
  __InputSSForSFun__/6(__UniqueOutportName__6__) -> InverterTvF_sfcn/6
  __InputSSForSFun__/7(__UniqueOutportName__7__) -> InverterTvF_sfcn/7
  InverterTvF_sfcn/1 -> __OutputSSForSFun__/1(__UniqueInportName__1__)
  InverterTvF_sfcn/2 -> __OutputSSForSFun__/2(__UniqueInportName__2__)
  InverterTvF_sfcn/3 -> __OutputSSForSFun__/3(__UniqueInportName__3__)
  InverterTvF_sfcn/4 -> __OutputSSForSFun__/4(__UniqueInportName__4__)
  __OutputSSForSFun__/1(Iu) -> Iu/1
  __OutputSSForSFun__/2(Iz) -> Iz/1
  __OutputSSForSFun__/3(Id) -> Id/1
  __OutputSSForSFun__/4(Vv) -> Vv/1

== system CRH2forBenchmark_Copy/InverterF/InverterTwF ==
  Tw1 : Inport
  Tw2 : Inport  Port=2
  Tw3 : Inport  Port=3
  Tw4 : Inport  Port=4
  Ic : Inport  Port=5
  U1 : Inport  Port=6
  U2 : Inport  Port=7
  InverterTwF_sfcn : S-Function  FunctionName=InverterTwF_sf  SFunctionModules=""  EnableBusSupport=off  mask{rtw_sf_name=InverterTwF_sf, showVar=off}
      mask prompts: rtw_sf_name "Simulink:masks:GenSFuncName_MP"; showVar "Simulink:masks:GenSFuncShowModuleList_MP"
      mask help: Simulink:masks:GenSFuncDesc_MD
      mask init: same as CRH2forBenchmark_Copy/DCU1/DCU1_sfcn
      settings: CopyFcn=|
      | if ~strcmp(get_param(gcb,'Linkstatus'),'none') && ...
      | ~strcmp(get_param(gcb,'Linkstatus'),'implicit')
      |   set_param(gcb,'LinkStatus','none');
      | end
      mask Help: eval('feval(''rtwprivate'',''rtwhelpview'',''rtw_sfcn_block'')');
      mask Display:
      | port_label('input',1,'Tw1');
      | port_label('input',2,'Tw2');
      | port_label('input',3,'Tw3');
      | port_label('input',4,'Tw4');
      | port_label('input',5,'Ic');
      | port_label('input',6,'U1');
      | port_label('input',7,'U2');
      | port_label('output',1,'Iu');
      | port_label('output',2,'Iz');
      | port_label('output',3,'Id');
      | port_label('output',4,'Vw');
  __InputSSForSFun__ : Subsystem
  __OutputSSForSFun__ : Subsystem
  Iu : Outport
  Iz : Outport  Port=2
  Id : Outport  Port=3
  Vw : Outport  Port=4
  wires:
  Tw1/1 -> __InputSSForSFun__/1(Tw1)
  Tw2/1 -> __InputSSForSFun__/2(Tw2)
  Tw3/1 -> __InputSSForSFun__/3(Tw3)
  Tw4/1 -> __InputSSForSFun__/4(Tw4)
  Ic/1 -> __InputSSForSFun__/5(Ic)
  U1/1 -> __InputSSForSFun__/6(U1)
  U2/1 -> __InputSSForSFun__/7(U2)
  __InputSSForSFun__/1(__UniqueOutportName__1__) -> InverterTwF_sfcn/1
  __InputSSForSFun__/2(__UniqueOutportName__2__) -> InverterTwF_sfcn/2
  __InputSSForSFun__/3(__UniqueOutportName__3__) -> InverterTwF_sfcn/3
  __InputSSForSFun__/4(__UniqueOutportName__4__) -> InverterTwF_sfcn/4
  __InputSSForSFun__/5(__UniqueOutportName__5__) -> InverterTwF_sfcn/5
  __InputSSForSFun__/6(__UniqueOutportName__6__) -> InverterTwF_sfcn/6
  __InputSSForSFun__/7(__UniqueOutportName__7__) -> InverterTwF_sfcn/7
  InverterTwF_sfcn/1 -> __OutputSSForSFun__/1(__UniqueInportName__1__)
  InverterTwF_sfcn/2 -> __OutputSSForSFun__/2(__UniqueInportName__2__)
  InverterTwF_sfcn/3 -> __OutputSSForSFun__/3(__UniqueInportName__3__)
  InverterTwF_sfcn/4 -> __OutputSSForSFun__/4(__UniqueInportName__4__)
  __OutputSSForSFun__/1(Iu) -> Iu/1
  __OutputSSForSFun__/2(Iz) -> Iz/1
  __OutputSSForSFun__/3(Id) -> Id/1
  __OutputSSForSFun__/4(Vw) -> Vw/1

== system CRH2forBenchmark_Copy/InverterF/Pulse ==
  note: PhaseA:1 to 4
      |
      | PhaseB:5 to 8
      |
      | PhaseC:9 to 12
  State : Inport
  Add : Sum
  Constant : Constant  Value=2
  Demux : Demux  Outputs=3
  Multiport Switch : MultiPortSwitch
  Multiport Switch1 : MultiPortSwitch
  Multiport Switch2 : MultiPortSwitch
  Mux : Mux  Inputs=3
  S =  Ud : Constant  Value=[1 1 0 0]
  S = - Ud : Constant  Value=[0 0 1 1]
  S = 0 : Constant  Value=[0 1 1 0]
  SVPWM : Outport
  wires:
  Add/1 -> Demux/1
  Multiport Switch1/1 -> Mux/2
  S = 0/1 -> Multiport Switch/3, Multiport Switch1/3, Multiport Switch2/3
  Demux/2 -> Multiport Switch1/1
  Demux/3 -> Multiport Switch2/1
  State/1 -> Add/1
  Constant/1 -> Add/2
  Mux/1 -> SVPWM/1
  Demux/1 -> Multiport Switch/1
  Multiport Switch2/1 -> Mux/3
  S =  Ud/1 -> Multiport Switch/4, Multiport Switch1/4, Multiport Switch2/4
  Multiport Switch/1 -> Mux/1
  S = - Ud/1 -> Multiport Switch1/2, Multiport Switch/2, Multiport Switch2/2

== system CRH2forBenchmark_Copy/InverterN/InverterTuN ==
  Tu1 : Inport
  Tu2 : Inport  Port=2
  Tu3 : Inport  Port=3
  Tu4 : Inport  Port=4
  Ia : Inport  Port=5
  U1 : Inport  Port=6
  U2 : Inport  Port=7
  InverterTuN_sfcn : S-Function  FunctionName=InverterTuN_sf  SFunctionModules=""  EnableBusSupport=off  mask{rtw_sf_name=InverterTuN_sf, showVar=off}
      mask prompts: rtw_sf_name "Simulink:masks:GenSFuncName_MP"; showVar "Simulink:masks:GenSFuncShowModuleList_MP"
      mask help: Simulink:masks:GenSFuncDesc_MD
      mask init: same as CRH2forBenchmark_Copy/DCU1/DCU1_sfcn
      settings: CopyFcn=|
      | if ~strcmp(get_param(gcb,'Linkstatus'),'none') && ...
      | ~strcmp(get_param(gcb,'Linkstatus'),'implicit')
      |   set_param(gcb,'LinkStatus','none');
      | end
      mask Help: eval('feval(''rtwprivate'',''rtwhelpview'',''rtw_sfcn_block'')');
      mask Display:
      | port_label('input',1,'Tu1');
      | port_label('input',2,'Tu2');
      | port_label('input',3,'Tu3');
      | port_label('input',4,'Tu4');
      | port_label('input',5,'Ia');
      | port_label('input',6,'U1');
      | port_label('input',7,'U2');
      | port_label('output',1,'Iu');
      | port_label('output',2,'Iz');
      | port_label('output',3,'Id');
      | port_label('output',4,'Vu');
  __InputSSForSFun__ : Subsystem
  __OutputSSForSFun__ : Subsystem
  Iu : Outport
  Iz : Outport  Port=2
  Id : Outport  Port=3
  Vu : Outport  Port=4
  wires:
  Tu1/1 -> __InputSSForSFun__/1(Tu1)
  Tu2/1 -> __InputSSForSFun__/2(Tu2)
  Tu3/1 -> __InputSSForSFun__/3(Tu3)
  Tu4/1 -> __InputSSForSFun__/4(Tu4)
  Ia/1 -> __InputSSForSFun__/5(Ia)
  U1/1 -> __InputSSForSFun__/6(U1)
  U2/1 -> __InputSSForSFun__/7(U2)
  __InputSSForSFun__/1(__UniqueOutportName__1__) -> InverterTuN_sfcn/1
  __InputSSForSFun__/2(__UniqueOutportName__2__) -> InverterTuN_sfcn/2
  __InputSSForSFun__/3(__UniqueOutportName__3__) -> InverterTuN_sfcn/3
  __InputSSForSFun__/4(__UniqueOutportName__4__) -> InverterTuN_sfcn/4
  __InputSSForSFun__/5(__UniqueOutportName__5__) -> InverterTuN_sfcn/5
  __InputSSForSFun__/6(__UniqueOutportName__6__) -> InverterTuN_sfcn/6
  __InputSSForSFun__/7(__UniqueOutportName__7__) -> InverterTuN_sfcn/7
  InverterTuN_sfcn/1 -> __OutputSSForSFun__/1(__UniqueInportName__1__)
  InverterTuN_sfcn/2 -> __OutputSSForSFun__/2(__UniqueInportName__2__)
  InverterTuN_sfcn/3 -> __OutputSSForSFun__/3(__UniqueInportName__3__)
  InverterTuN_sfcn/4 -> __OutputSSForSFun__/4(__UniqueInportName__4__)
  __OutputSSForSFun__/1(Iu) -> Iu/1
  __OutputSSForSFun__/2(Iz) -> Iz/1
  __OutputSSForSFun__/3(Id) -> Id/1
  __OutputSSForSFun__/4(Vu) -> Vu/1

== system CRH2forBenchmark_Copy/InverterN/InverterTvN ==
  Tv1 : Inport
  Tv2 : Inport  Port=2
  Tv3 : Inport  Port=3
  Tv4 : Inport  Port=4
  Ib : Inport  Port=5
  U1 : Inport  Port=6
  U2 : Inport  Port=7
  InverterTvN_sfcn : S-Function  FunctionName=InverterTvN_sf  SFunctionModules=""  EnableBusSupport=off  mask{rtw_sf_name=InverterTvN_sf, showVar=off}
      mask prompts: rtw_sf_name "Simulink:masks:GenSFuncName_MP"; showVar "Simulink:masks:GenSFuncShowModuleList_MP"
      mask help: Simulink:masks:GenSFuncDesc_MD
      mask init: same as CRH2forBenchmark_Copy/DCU1/DCU1_sfcn
      settings: CopyFcn=|
      | if ~strcmp(get_param(gcb,'Linkstatus'),'none') && ...
      | ~strcmp(get_param(gcb,'Linkstatus'),'implicit')
      |   set_param(gcb,'LinkStatus','none');
      | end
      mask Help: eval('feval(''rtwprivate'',''rtwhelpview'',''rtw_sfcn_block'')');
      mask Display:
      | port_label('input',1,'Tv1');
      | port_label('input',2,'Tv2');
      | port_label('input',3,'Tv3');
      | port_label('input',4,'Tv4');
      | port_label('input',5,'Ib');
      | port_label('input',6,'U1');
      | port_label('input',7,'U2');
      | port_label('output',1,'Iu');
      | port_label('output',2,'Iz');
      | port_label('output',3,'Id');
      | port_label('output',4,'Vv');
  __InputSSForSFun__ : Subsystem
  __OutputSSForSFun__ : Subsystem
  Iu : Outport
  Iz : Outport  Port=2
  Id : Outport  Port=3
  Vv : Outport  Port=4
  wires:
  Tv1/1 -> __InputSSForSFun__/1(Tv1)
  Tv2/1 -> __InputSSForSFun__/2(Tv2)
  Tv3/1 -> __InputSSForSFun__/3(Tv3)
  Tv4/1 -> __InputSSForSFun__/4(Tv4)
  Ib/1 -> __InputSSForSFun__/5(Ib)
  U1/1 -> __InputSSForSFun__/6(U1)
  U2/1 -> __InputSSForSFun__/7(U2)
  __InputSSForSFun__/1(__UniqueOutportName__1__) -> InverterTvN_sfcn/1
  __InputSSForSFun__/2(__UniqueOutportName__2__) -> InverterTvN_sfcn/2
  __InputSSForSFun__/3(__UniqueOutportName__3__) -> InverterTvN_sfcn/3
  __InputSSForSFun__/4(__UniqueOutportName__4__) -> InverterTvN_sfcn/4
  __InputSSForSFun__/5(__UniqueOutportName__5__) -> InverterTvN_sfcn/5
  __InputSSForSFun__/6(__UniqueOutportName__6__) -> InverterTvN_sfcn/6
  __InputSSForSFun__/7(__UniqueOutportName__7__) -> InverterTvN_sfcn/7
  InverterTvN_sfcn/1 -> __OutputSSForSFun__/1(__UniqueInportName__1__)
  InverterTvN_sfcn/2 -> __OutputSSForSFun__/2(__UniqueInportName__2__)
  InverterTvN_sfcn/3 -> __OutputSSForSFun__/3(__UniqueInportName__3__)
  InverterTvN_sfcn/4 -> __OutputSSForSFun__/4(__UniqueInportName__4__)
  __OutputSSForSFun__/1(Iu) -> Iu/1
  __OutputSSForSFun__/2(Iz) -> Iz/1
  __OutputSSForSFun__/3(Id) -> Id/1
  __OutputSSForSFun__/4(Vv) -> Vv/1

== system CRH2forBenchmark_Copy/InverterN/InverterTwN ==
  Tw1 : Inport
  Tw2 : Inport  Port=2
  Tw3 : Inport  Port=3
  Tw4 : Inport  Port=4
  Ic : Inport  Port=5
  U1 : Inport  Port=6
  U2 : Inport  Port=7
  InverterTwN_sfcn : S-Function  FunctionName=InverterTwN_sf  SFunctionModules=""  EnableBusSupport=off  mask{rtw_sf_name=InverterTwN_sf, showVar=off}
      mask prompts: rtw_sf_name "Simulink:masks:GenSFuncName_MP"; showVar "Simulink:masks:GenSFuncShowModuleList_MP"
      mask help: Simulink:masks:GenSFuncDesc_MD
      mask init: same as CRH2forBenchmark_Copy/DCU1/DCU1_sfcn
      settings: CopyFcn=|
      | if ~strcmp(get_param(gcb,'Linkstatus'),'none') && ...
      | ~strcmp(get_param(gcb,'Linkstatus'),'implicit')
      |   set_param(gcb,'LinkStatus','none');
      | end
      mask Help: eval('feval(''rtwprivate'',''rtwhelpview'',''rtw_sfcn_block'')');
      mask Display:
      | port_label('input',1,'Tw1');
      | port_label('input',2,'Tw2');
      | port_label('input',3,'Tw3');
      | port_label('input',4,'Tw4');
      | port_label('input',5,'Ic');
      | port_label('input',6,'U1');
      | port_label('input',7,'U2');
      | port_label('output',1,'Iu');
      | port_label('output',2,'Iz');
      | port_label('output',3,'Id');
      | port_label('output',4,'Vw');
  __InputSSForSFun__ : Subsystem
  __OutputSSForSFun__ : Subsystem
  Iu : Outport
  Iz : Outport  Port=2
  Id : Outport  Port=3
  Vw : Outport  Port=4
  wires:
  Tw1/1 -> __InputSSForSFun__/1(Tw1)
  Tw2/1 -> __InputSSForSFun__/2(Tw2)
  Tw3/1 -> __InputSSForSFun__/3(Tw3)
  Tw4/1 -> __InputSSForSFun__/4(Tw4)
  Ic/1 -> __InputSSForSFun__/5(Ic)
  U1/1 -> __InputSSForSFun__/6(U1)
  U2/1 -> __InputSSForSFun__/7(U2)
  __InputSSForSFun__/1(__UniqueOutportName__1__) -> InverterTwN_sfcn/1
  __InputSSForSFun__/2(__UniqueOutportName__2__) -> InverterTwN_sfcn/2
  __InputSSForSFun__/3(__UniqueOutportName__3__) -> InverterTwN_sfcn/3
  __InputSSForSFun__/4(__UniqueOutportName__4__) -> InverterTwN_sfcn/4
  __InputSSForSFun__/5(__UniqueOutportName__5__) -> InverterTwN_sfcn/5
  __InputSSForSFun__/6(__UniqueOutportName__6__) -> InverterTwN_sfcn/6
  __InputSSForSFun__/7(__UniqueOutportName__7__) -> InverterTwN_sfcn/7
  InverterTwN_sfcn/1 -> __OutputSSForSFun__/1(__UniqueInportName__1__)
  InverterTwN_sfcn/2 -> __OutputSSForSFun__/2(__UniqueInportName__2__)
  InverterTwN_sfcn/3 -> __OutputSSForSFun__/3(__UniqueInportName__3__)
  InverterTwN_sfcn/4 -> __OutputSSForSFun__/4(__UniqueInportName__4__)
  __OutputSSForSFun__/1(Iu) -> Iu/1
  __OutputSSForSFun__/2(Iz) -> Iz/1
  __OutputSSForSFun__/3(Id) -> Id/1
  __OutputSSForSFun__/4(Vw) -> Vw/1

== system CRH2forBenchmark_Copy/InverterN/Pulse ==
  note: PhaseA:1 to 4
      |
      | PhaseB:5 to 8
      |
      | PhaseC:9 to 12
  State : Inport
  Add : Sum
  Constant : Constant  Value=2
  Demux : Demux  Outputs=3
  Multiport Switch : MultiPortSwitch
  Multiport Switch1 : MultiPortSwitch
  Multiport Switch2 : MultiPortSwitch
  Mux : Mux  Inputs=3
  S =  Ud : Constant  Value=[1 1 0 0]
  S = - Ud : Constant  Value=[0 0 1 1]
  S = 0 : Constant  Value=[0 1 1 0]
  SVPWM : Outport
  wires:
  S = - Ud/1 -> Multiport Switch2/2, Multiport Switch/2, Multiport Switch1/2
  Multiport Switch/1 -> Mux/1
  S =  Ud/1 -> Multiport Switch2/4, Multiport Switch1/4, Multiport Switch/4
  Multiport Switch2/1 -> Mux/3
  Demux/1 -> Multiport Switch/1
  Mux/1 -> SVPWM/1
  Constant/1 -> Add/2
  State/1 -> Add/1
  Demux/3 -> Multiport Switch2/1
  Demux/2 -> Multiport Switch1/1
  S = 0/1 -> Multiport Switch2/3, Multiport Switch1/3, Multiport Switch/3
  Multiport Switch1/1 -> Mux/2
  Add/1 -> Demux/1

== system CRH2forBenchmark_Copy/Machine model/Normal ModelF ==
  Ua : Inport
  Ub : Inport  Port=2
  Uc : Inport  Port=3
  TL : Inport  Port=4
  MeasurementF : Subsystem  mask{sfcnParam1=J, sfcnParam2=Lm, sfcnParam3=np}
      mask prompts: sfcnParam1 "J:"; sfcnParam2 "Lm:"; sfcnParam3 "np:"
      mask help: Simulink:masks:GenSFuncDesc_MD
      mask Help: eval('feval(''rtwprivate'',''rtwhelpview'',''rtw_sfcn_block'')');
  MotorSubsystem1F : Subsystem
  MotorSubsystem2F : Subsystem
  MotorSubsystem3F : Subsystem
  MotorSubsystemF : Subsystem
  r2sF : Subsystem
      mask help: Simulink:masks:GenSFuncDesc_MD
      mask Help: eval('feval(''rtwprivate'',''rtwhelpview'',''rtw_sfcn_block'')');
  Te0 : Outport
  Isabc0 : Outport  Port=2
  w : Outport  Port=3
  wires:
  MeasurementF/3(Isabc) -> Isabc0/1
  MotorSubsystem2F/2(ψrα) -> MotorSubsystem3F/2(ψrα), MotorSubsystemF/1(ψrα)
  MotorSubsystem1F/2(ψsβ) -> MotorSubsystem3F/1(ψsβ)
  MotorSubsystem2F/1(irα) -> MeasurementF/3(irα)
  MeasurementF/1(Te) -> Te0/1
  TL/1 -> MeasurementF/5(TL)
  MotorSubsystemF/2(ψsα) -> MotorSubsystem2F/1(ψsα)
  r2sF/1(Usα) -> MotorSubsystemF/2(Usα)
  MotorSubsystem3F/2(ψrβ) -> MotorSubsystem1F/1(ψrβ), MotorSubsystem2F/2(ψrβ)
  MotorSubsystemF/1(isα) -> MeasurementF/1(isα)
  r2sF/2(Usβ) -> MotorSubsystem1F/2(Usβ)
  MotorSubsystem3F/1(irβ) -> MeasurementF/4(irβ)
  MeasurementF/2(ω) -> MotorSubsystem2F/3(ω), MotorSubsystem3F/3(ω), w/1
  MotorSubsystem1F/1(isβ) -> MeasurementF/2(isβ)
  Uc/1 -> r2sF/3(Uc)
  Ub/1 -> r2sF/2(Ub)
  Ua/1 -> r2sF/1(Ua)

== system CRH2forBenchmark_Copy/Machine model1/Normal ModelN ==
  Ua : Inport
  Ub : Inport  Port=2
  Uc : Inport  Port=3
  TL : Inport  Port=4
  MeasurementN : Subsystem  mask{sfcnParam1=J, sfcnParam2=Lm, sfcnParam3=np}
      mask prompts: sfcnParam1 "J:"; sfcnParam2 "Lm:"; sfcnParam3 "np:"
      mask help: Simulink:masks:GenSFuncDesc_MD
      mask Help: eval('feval(''rtwprivate'',''rtwhelpview'',''rtw_sfcn_block'')');
  MotorSubsystem1N : Subsystem
  MotorSubsystem2N : Subsystem
  MotorSubsystem3N : Subsystem
  MotorSubsystemN : Subsystem
  r2sN : Subsystem
      mask help: Simulink:masks:GenSFuncDesc_MD
      mask Help: eval('feval(''rtwprivate'',''rtwhelpview'',''rtw_sfcn_block'')');
  Te0 : Outport
  Isabc0 : Outport  Port=2
  w : Outport  Port=3
  wires:
  MeasurementN/3(Isabc) -> Isabc0/1
  MotorSubsystem2N/2(ψrα) -> MotorSubsystem3N/2(ψrα), MotorSubsystemN/1(ψrα)
  MotorSubsystem1N/2(ψsβ) -> MotorSubsystem3N/1(ψsβ)
  MotorSubsystem2N/1(irα) -> MeasurementN/3(irα)
  MeasurementN/1(Te) -> Te0/1
  TL/1 -> MeasurementN/5(TL)
  MotorSubsystemN/2(ψsα) -> MotorSubsystem2N/1(ψsα)
  r2sN/1(Usα) -> MotorSubsystemN/2(Usα)
  MotorSubsystem3N/2(ψrβ) -> MotorSubsystem1N/1(ψrβ), MotorSubsystem2N/2(ψrβ)
  MotorSubsystemN/1(isα) -> MeasurementN/1(isα)
  r2sN/2(Usβ) -> MotorSubsystem1N/2(Usβ)
  MotorSubsystem3N/1(irβ) -> MeasurementN/4(irβ)
  MeasurementN/2(ω) -> MotorSubsystem2N/3(ω), MotorSubsystem3N/3(ω), w/1
  MotorSubsystem1N/1(isβ) -> MeasurementN/2(isβ)
  Uc/1 -> r2sN/3(Uc)
  Ub/1 -> r2sN/2(Ub)
  Ua/1 -> r2sN/1(Ua)

== system CRH2forBenchmark_Copy/Benchmark/CFI1/Subsystem2 ==
  Nomal : Inport
  Outside Signal1 : Inport  Port=2
  Band-Limited White Noise : simulink/Sources/Band-Limited White Noise  Cov=NoiseFault(1)  Ts=NoiseFault(2)  seed=NoiseFault(3)
  Subsystem : Subsystem
  Subsystem1 : Subsystem  mask{sfcnParam1=AddMux, sfcnParam2=ContantofPassiveDevice, sfcnParam3=FaultInjectionTime, sfcnParam4=FaultType, sfcnParam5=NoiseSelec, sfcnParam6=PerformanceDegradationValue}
      mask prompts: sfcnParam1 "AddMux:"; sfcnParam2 "ContantofPassiveDevice:"; sfcnParam3 "FaultInjectionTime:"; sfcnParam4 "FaultType:"; sfcnParam5 "NoiseSelec:"; sfcnParam6 "PerformanceDegradationValue:"
      mask help: Simulink:masks:GenSFuncDesc_MD
      mask Help: eval('feval(''rtwprivate'',''rtwhelpview'',''rtw_sfcn_block'')');
  Out : Outport
  tag scope: BandLimitedWhiteNoiseCFI1=global, PeriodicSignalsCFI1=global
  wires:
  Subsystem/1(Periodic Signals) -> [PeriodicSignalsCFI1]
  Band-Limited White Noise/1 -> [BandLimitedWhiteNoiseCFI1]
  Nomal/1 -> Subsystem1/1(Nomal)
  Outside Signal1/1 -> Subsystem1/2(Outside Signal1)
  Subsystem1/1(Out) -> Out/1

== system CRH2forBenchmark_Copy/Benchmark/CFI2/Subsystem2 ==
  Nomal : Inport
  Outside Signal1 : Inport  Port=2
  Band-Limited White Noise : simulink/Sources/Band-Limited White Noise  Cov=NoiseFault(1)  Ts=NoiseFault(2)  seed=NoiseFault(3)
  Subsystem : Subsystem
  Subsystem1 : Subsystem  mask{sfcnParam1=AddMux, sfcnParam2=ContantofPassiveDevice, sfcnParam3=FaultInjectionTime, sfcnParam4=FaultType, sfcnParam5=NoiseSelec, sfcnParam6=PerformanceDegradationValue}
      mask prompts: sfcnParam1 "AddMux:"; sfcnParam2 "ContantofPassiveDevice:"; sfcnParam3 "FaultInjectionTime:"; sfcnParam4 "FaultType:"; sfcnParam5 "NoiseSelec:"; sfcnParam6 "PerformanceDegradationValue:"
      mask help: Simulink:masks:GenSFuncDesc_MD
      mask Help: eval('feval(''rtwprivate'',''rtwhelpview'',''rtw_sfcn_block'')');
  Out : Outport
  tag scope: BandLimitedWhiteNoiseCFI2=global, PeriodicSignalsCFI2=global
  wires:
  Subsystem/1(Periodic Signals) -> [PeriodicSignalsCFI2]
  Band-Limited White Noise/1 -> [BandLimitedWhiteNoiseCFI2]
  Nomal/1 -> Subsystem1/1(Nomal)
  Outside Signal1/1 -> Subsystem1/2(Outside Signal1)
  Subsystem1/1(Out) -> Out/1

== system CRH2forBenchmark_Copy/Benchmark/MFI1/MFI1 ==
  Nomal : Inport
  Outside Signal1 : Inport  Port=2
  "MFI " : Subsystem
  Out : Outport
  wires:
  "MFI "/1(Out) -> Out/1
  Outside Signal1/1 -> "MFI "/2(OutsideSignal)
  Nomal/1 -> "MFI "/1(Normal)

== system CRH2forBenchmark_Copy/Benchmark/MFI1/MFI2 ==
  Nomal : Inport
  Outside Signal1 : Inport  Port=2
  "MFI " : Subsystem
  Out : Outport
  wires:
  Nomal/1 -> "MFI "/1(Normal)
  "MFI "/1(Out) -> Out/1
  Outside Signal1/1 -> "MFI "/2(OutsideSignal)

== system CRH2forBenchmark_Copy/Benchmark/MFI1/MFI3 ==
  Nomal : Inport
  Outside Signal1 : Inport  Port=2
  "MFI " : Subsystem
  Out : Outport
  wires:
  "MFI "/1(Out) -> Out/1
  Nomal/1 -> "MFI "/1(Normal)
  Outside Signal1/1 -> "MFI "/2(OutsideSignal)

== system CRH2forBenchmark_Copy/Benchmark/MFI1/MFI4 ==
  Nomal : Inport
  Outside Signal1 : Inport  Port=2
  "MFI " : Subsystem
  Out : Outport
  wires:
  "MFI "/1(Out) -> Out/1
  Outside Signal1/1 -> "MFI "/2(OutsideSignal)
  Nomal/1 -> "MFI "/1(Normal)

== system CRH2forBenchmark_Copy/Benchmark/MFI1/MFI5 ==
  Nomal : Inport
  Outside Signal1 : Inport  Port=2
  "MFI " : Subsystem
  Out : Outport
  wires:
  Nomal/1 -> "MFI "/1(Normal)
  "MFI "/1(Out) -> Out/1
  Outside Signal1/1 -> "MFI "/2(OutsideSignal)

== system CRH2forBenchmark_Copy/Benchmark/MFI1/MFI6 ==
  Nomal : Inport
  Outside Signal1 : Inport  Port=2
  "MFI " : Subsystem
  Out : Outport
  wires:
  Nomal/1 -> "MFI "/1(Normal)
  "MFI "/1(Out) -> Out/1
  Outside Signal1/1 -> "MFI "/2(OutsideSignal)

== system CRH2forBenchmark_Copy/Benchmark/SFI1/Subsystem ==
  Normal : Inport
  Outside Signal : Inport  Port=2
  Band-Limited White Noise : simulink/Sources/Band-Limited White Noise  Cov=NoiseFault(1)  Ts=NoiseFault(2)  seed=NoiseFault(3)
  Pulse Generator : DiscretePulseGenerator  PulseType=Time based  Amplitude=PeriodicFault(1)  Period=PeriodicFault(2)  PulseWidth=PeriodicFault(3)
  SFI1 : Subsystem  mask{sfcnParam1=AddMux, sfcnParam2=Comp_ConV, sfcnParam3=DriftFault, sfcnParam4=FaultCont, sfcnParam5=FaultInjectionTime, sfcnParam6=FaultType, sfcnParam7=NoiseSelec, sfcnParam8=ShockGain, sfcnParam9=Variance}
      mask prompts: sfcnParam1 "AddMux:"; sfcnParam2 "Comp_ConV:"; sfcnParam3 "DriftFault:"; sfcnParam4 "FaultCont:"; sfcnParam5 "FaultInjectionTime:"; sfcnParam6 "FaultType:"; sfcnParam7 "NoiseSelec:"; sfcnParam8 "ShockGain:"; sfcnParam9 "Variance:"
      mask help: Simulink:masks:GenSFuncDesc_MD
      mask Help: eval('feval(''rtwprivate'',''rtwhelpview'',''rtw_sfcn_block'')');
  Out : Outport
  tag scope: BandLimitedWhiteNoiseSFI1=global, PulseGeneratorSFI1=global
  wires:
  Band-Limited White Noise/1 -> [BandLimitedWhiteNoiseSFI1]
  Pulse Generator/1 -> [PulseGeneratorSFI1]
  Normal/1 -> SFI1/1(Nomal)
  Outside Signal/1 -> SFI1/2(Outside Signal)
  SFI1/1(Out) -> Out/1
